simulink library "drg"  (Simulink 8.1)
settings: Solver=ode1  StartTime=0.0  StopTime=Inf  FixedStep=0.001  RelTol=1e-3
PostLoadFcn:
  | , if any(exist('dsrtsu_mdlpostloadfcn', 'file') == [2, 3, 6]), try dsrtsu_mdlpostloadfcn('Execute', bdroot); catch fprintf('Error in PostLoadFcn (dsrtsu_mdlpostloadfcn) for model "%s":\n %s\n', bdroot, lasterr); end, end,
undefined symbols (not defined in the file or in its folder): ZERO_FLOAT
libraries: dbt x1, dnb x1
settings Model: DSRTSU_INTERNAL_RTI_VER=450  DSRTSU_INTERNAL_RTI_TYPE=rti1401  RTICANMMDATA=struct('GeneralSetupData',struct('modelroot','D:\ELN150201_TAIWAN\trunk\AdasDragon\software\sw_development\arch\app\acc','generalsettings',struct('filesettings',struct('destfolder',struct('Name','RTICANMM_FILES','Check',1),'buildfolder',struct('Name','.','Check',1),'AbsDestfolder',struct('Name','D:\ELN150201_TAIWAN\trunk\AdasDragon\software\sw_development\arch\app\acc\RTICANMM_FILES'),'AbsBuildfolder',struct('Name','D:\ELN150201_TAIWAN\trunk\AdasDragon\software\sw_development\arch\app\acc'))),'options',struct('addpaths',1,'rmpaths',1,'addtrcexclusion',logical(1),'cannavigator',struct('checkmonitoring',0),'show_usrtrc',0,'use_usrtrc',0),'advanced',struct('options',[1 1 1 1 1 1 1 1 1 1 1 1 1 1 1 1 1 1 1 1 1 1 1 1 1 1 1 1 1 1 1 1 1 1 1 1 1 1 1 1 1 1 1 1 1 1 1 1 1 1 1 1 1 1 1 1 1 1 1 1 1 1 1 1 1 1 1 1 1 1 1 1 1 1 1 1 1 1 1 1 1 1 1 1 1 1 1 1 1 1 1 1 1 1 1 1 1 1 1 1]),'MPSetup',{{}},'modelname','drd','block','drd'))  DSRTSU_INTERNAL_RTIFPGA=40  Creator=AT015555  LastModifiedBy=AT015555

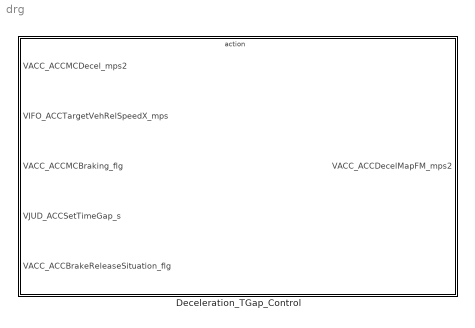
== system drg ==
  Deceleration_TGap_Control : Subsystem  TreatAsAtomicUnit=on

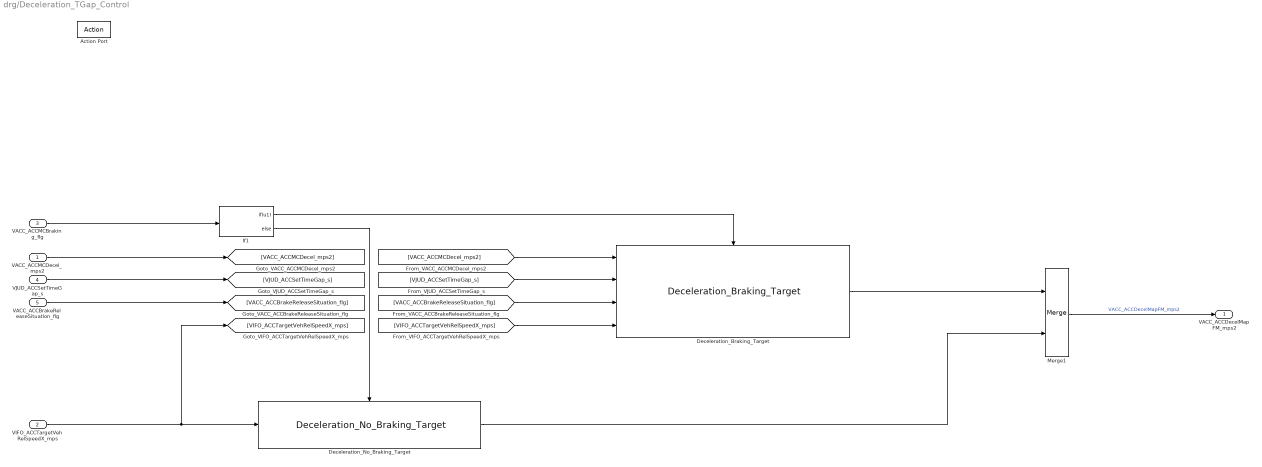
== system drg/Deceleration_TGap_Control ==
  VACC_ACCMCDecel_mps2 : Inport
  VIFO_ACCTargetVehRelSpeedX_mps : Inport  Port=2
  VACC_ACCMCBraking_flg : Inport  Port=3
  VJUD_ACCSetTimeGap_s : Inport  Port=4
  VACC_ACCBrakeReleaseSituation_flg : Inport  Port=5
  Action Port : ActionPort
  Deceleration_Braking_Target : dbt/Deceleration_Braking_Target
  Deceleration_No_Braking_Target : dnb/Deceleration_No_Braking_Target
  If1 : If  IfExpression=u1
  Merge1 : Merge
  VACC_ACCDecelMapFM_mps2 : Outport  OutputWhenDisabled=reset  InitialOutput=ZERO_FLOAT
  wires:
  VACC_ACCBrakeReleaseSituation_flg/1 -> [VACC_ACCBrakeReleaseSituation_flg]
  [VACC_ACCBrakeReleaseSituation_flg] -> Deceleration_Braking_Target/3
  [VJUD_ACCSetTimeGap_s] -> Deceleration_Braking_Target/2
  VJUD_ACCSetTimeGap_s/1 -> [VJUD_ACCSetTimeGap_s]
  VACC_ACCMCBraking_flg/1 -> If1/1
  Deceleration_Braking_Target/1 -> Merge1/1
  [VACC_ACCMCDecel_mps2] -> Deceleration_Braking_Target/1
  [VIFO_ACCTargetVehRelSpeedX_mps] -> Deceleration_Braking_Target/4
  If1/1 -> Deceleration_Braking_Target/Action
  If1/2 -> Deceleration_No_Braking_Target/Action
  Deceleration_No_Braking_Target/1 -> Merge1/2
  Merge1/1 -> VACC_ACCDecelMapFM_mps2/1  "VACC_ACCDecelMapFM_mps2"
  VACC_ACCMCDecel_mps2/1 -> [VACC_ACCMCDecel_mps2]
  VIFO_ACCTargetVehRelSpeedX_mps/1 -> [VIFO_ACCTargetVehRelSpeedX_mps], Deceleration_No_Braking_Target/1
